simulink model "powerassignment"  (R2019a)
settings: Solver=VariableStepAuto  StartTime=0.0  StopTime=3.0  RelTol=1e-3
libraries: powerlib x17
settings Model: Creator=Leah  LastModifiedBy=Leah

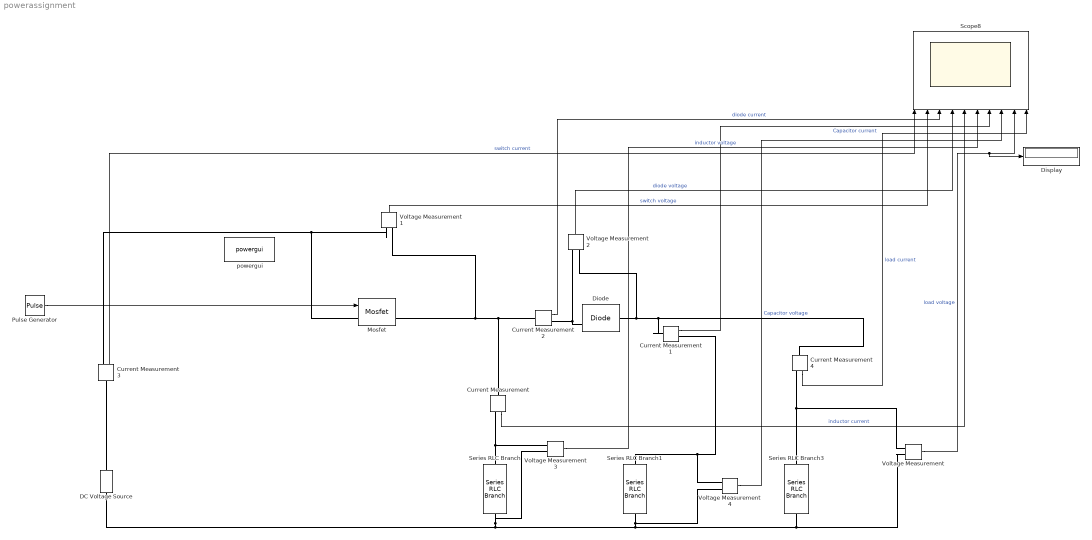
== system powerassignment ==
  Current Measurement{,1..4} (5 alike) : powerlib/Measurements/Current Measurement  PhasorSimulation=off  OutputType=Complex  PSBequivalent=0
      settings: SourceProductName=Simscape Electrical
  DC Voltage Source : powerlib/Electrical Sources/DC Voltage Source  Amplitude=42  Measurements=None
      settings: SourceProductName=Simscape Electrical
  Diode : powerlib/Power Electronics/Diode  Ron=2.1  Lon=0  Vf=0  IC=0  UseSnubber=0  Rs=0.005  Cs=0  Measurements=on
      settings: SourceProductName=Simscape Electrical
  Display : Display
  Mosfet : powerlib/Power Electronics/Mosfet  Ron=0  Lon=0  Rd=0.00  Vfd=0.0  IC=0  Rs=1e5  Cs=0  Measurements=on
      settings: SourceProductName=Simscape Electrical
  Pulse Generator : DiscretePulseGenerator  PulseType=Time based  Period=5e-5  PulseWidth=46.15
  Scope8 : Scope  NumInputPorts=10
  Series RLC Branch : powerlib/Elements/Series RLC Branch  LConnTagsString=__new0  RConnTagsString=__new0  BranchType=L  Resistance=1  Inductance=2.324e-5  SetiL0=off  InitialCurrent=0  Capacitance=1e-6  Setx0=off  InitialVoltage=0  Measurements=Branch voltage and current
      settings: SourceProductName=Simscape Electrical
  Series RLC Branch1 : powerlib/Elements/Series RLC Branch  LConnTagsString=__new0  RConnTagsString=__new0  BranchType=C  Resistance=1  Inductance=1e-3  SetiL0=off  InitialCurrent=0  Capacitance=1.515e-4  Setx0=off  InitialVoltage=0  Measurements=Branch voltage and current
      settings: SourceProductName=Simscape Electrical
  Series RLC Branch3 : powerlib/Elements/Series RLC Branch  LConnTagsString=__new0  RConnTagsString=__new0  BranchType=R  Resistance=9  Inductance=1e-3  SetiL0=off  InitialCurrent=0  Capacitance=1e-6  Setx0=off  InitialVoltage=0  Measurements=None
      settings: SourceProductName=Simscape Electrical
  Voltage Measurement : powerlib/Measurements/Voltage Measurement  PhasorSimulation=off  OutputType=Magnitude  PSBequivalent=0
      settings: SourceProductName=Simscape Electrical
  Voltage Measurement{1..4} (4 alike) : powerlib/Measurements/Voltage Measurement  PhasorSimulation=off  OutputType=Complex  PSBequivalent=0
      settings: SourceProductName=Simscape Electrical
  powergui : powerlib/powergui  Priority=1  SimulationMode=Continuous  SampleTime=50e-6  frequency=60  Iterations=50  frequencyindice=0  Pbase=100e6  ErrMax=1e-4  UnitsV=kV  UnitsW=MW  buscounter=0  FunctionMessages=off  echomessages=off  EnableUseOfTLC=off  CurrentSourceSwitches=off  DisableSnubberDevices=off  DisableRonSwitches=off  DisableVfSwitches=off  DisplayEquations=off  AutomaticDiscreteSolvers=off  SolverType=Tustin/Backward Euler (TBE)  Interpol=off  ExternalGateDelay=off  methode=off  Ts=100  x0status=blocks  SPID=on  SwTol=0  HookPort=off  NonlinearTolerance=0  nMaxIteration=15  ContinueOnMaxIteration=off  RestoreLinks=warning  ResistiveCurrentMeasurement=off  Frange=[0:2:500]  Ylog=off  Xlog=on  ShowGrid=off  save=off  variable=ZData  structure=0  ZoomFFT=off  StartTime=0.0  cycles=1  DisplayStyle=1  fundamental=60  FreqAxis=off  MaxFrequency=1000  frequencyindicesteady=1  RmsSteady=1  display=off
      settings: SourceProductName=Simscape Electrical
  wires:
  Pulse Generator/1 -> Mosfet/1
  Voltage Measurement/1 -> Scope8/9, Display/1  "load voltage"
  Voltage Measurement3/1 -> Scope8/6  "inductor voltage"
  Current Measurement/1 -> Scope8/5  "inductor current"
  Voltage Measurement2/1 -> Scope8/4  "diode voltage"
  Current Measurement2/1 -> Scope8/3  "diode current"
  Voltage Measurement1/1 -> Scope8/2  "switch voltage"
  Current Measurement3/1 -> Scope8/1  "switch current"
  Voltage Measurement4/1 -> Scope8/8  "Capacitor voltage"
  Current Measurement1/1 -> Scope8/7  "Capacitor current"
  Current Measurement4/1 -> Scope8/10  "load current"
  connections:
  Current Measurement1/LConn1 -- Voltage Measurement2/LConn2 -- Diode/LConn1 -- Current Measurement4/LConn1
  Current Measurement/RConn1 -- Voltage Measurement3/LConn1 -- Series RLC Branch/LConn1
  Current Measurement3/LConn1 -- DC Voltage Source/RConn1
  Voltage Measurement2/LConn1 -- Diode/RConn1 -- Current Measurement2/RConn1
  Current Measurement3/RConn1 -- Mosfet/LConn1 -- Voltage Measurement1/LConn1
  Voltage Measurement4/LConn2 -- Series RLC Branch1/RConn1 -- Series RLC Branch3/RConn1 -- Voltage Measurement/LConn2 -- DC Voltage Source/LConn1 -- Voltage Measurement3/LConn2 -- Series RLC Branch/RConn1
  Voltage Measurement1/LConn2 -- Current Measurement/LConn1 -- Current Measurement2/LConn1 -- Mosfet/RConn1
  Voltage Measurement4/LConn1 -- Series RLC Branch1/LConn1 -- Current Measurement1/RConn1
  Series RLC Branch3/LConn1 -- Current Measurement4/RConn1 -- Voltage Measurement/LConn1
